simulink model "Q5_RMS"  (R2017b)
settings: Solver=VariableStepAuto  StartTime=0.0  StopTime=1000  RelTol=1e-3
libraries: dspstat3 x3
settings Model: Creator=YSNsec  LastModifiedBy=YSNsec
settings DataIOCC: ReturnWorkspaceOutputs=on
settings DebuggingCC: SFMachineParentedDataDiag=error
settings SFSimCC: SimUseLocalCustomCode=on
settings RTWCC: RTWUseLocalCustomCode=on

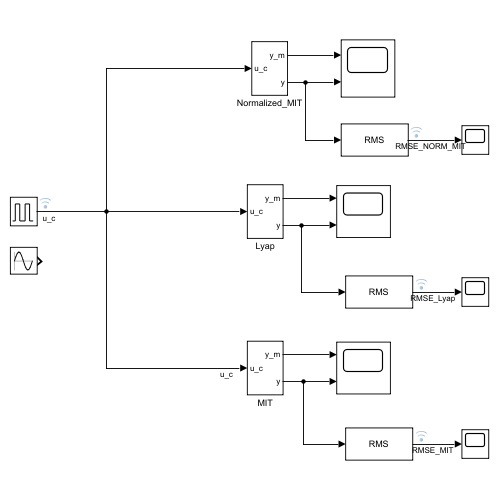
[thumbnail: Simulink's stored preview of the top-level diagram]
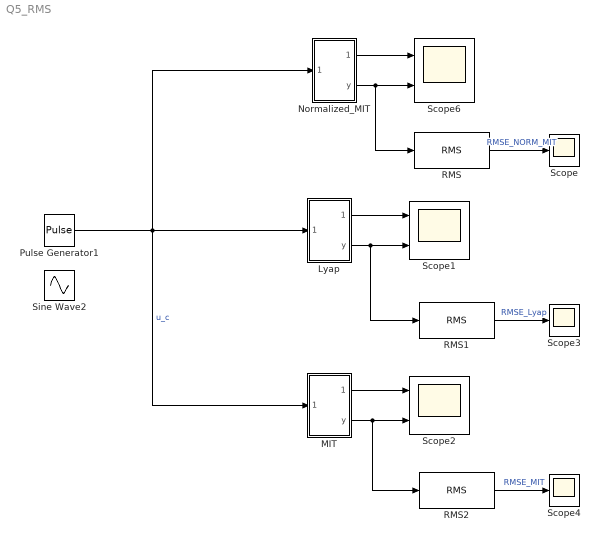
== system Q5_RMS ==
  Lyap : Subsystem
  MIT : Subsystem
  Normalized_MIT : Subsystem
  Pulse Generator1 : DiscretePulseGenerator  PulseType=Time based  Amplitude=10  Period=200  PulseWidth=50
  RMS : dspstat3/RMS  run=off  directionMode=Entire input  dimension=1  InputProcessing=Columns as channels (frame based)  reset_popup=None
  RMS1 : dspstat3/RMS  run=off  directionMode=Entire input  dimension=1  InputProcessing=Columns as channels (frame based)  reset_popup=None
  RMS2 : dspstat3/RMS  run=off  directionMode=Entire input  dimension=1  InputProcessing=Columns as channels (frame based)  reset_popup=None
  Scope : Scope
  Scope1 : Scope  NumInputPorts=2
  Scope2 : Scope  NumInputPorts=2
  Scope3 : Scope
  Scope4 : Scope
  Scope6 : Scope  NumInputPorts=2
  Sine Wave2 : Sin  Amplitude=10  Frequency=0.01  SampleTime=0
  wires:
  Normalized_MIT/1(y_m) -> Scope6/1
  Normalized_MIT/2(y) -> RMS/1, Scope6/2
  Lyap/1(y_m) -> Scope1/1
  Pulse Generator1/1 -> MIT/1(u_c), Lyap/1(u_c), Normalized_MIT/1(u_c)  "u_c"
  MIT/1(y_m) -> Scope2/1
  RMS/1 -> Scope/1  "RMSE_NORM_MIT"
  RMS1/1 -> Scope3/1  "RMSE_Lyap"
  Lyap/2(y) -> RMS1/1, Scope1/2
  RMS2/1 -> Scope4/1  "RMSE_MIT"
  MIT/2(y) -> RMS2/1, Scope2/2

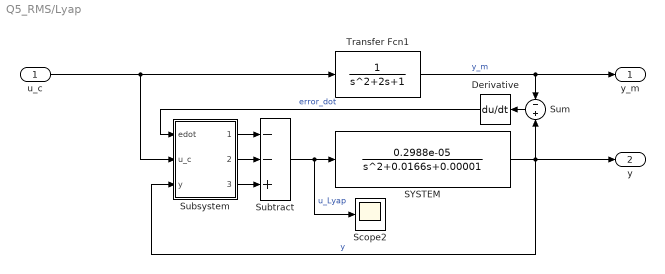
== system Q5_RMS/Lyap ==
  u_c : Inport
  Derivative : Derivative
  SYSTEM : TransferFcn  Numerator=0.2988e-05  Denominator=[1 0.0166 0.00001]
  Scope2 : Scope
  Subsystem : Subsystem
  Subtract : Sum  Inputs=--+
  Sum : Sum  Inputs=-|+
  Transfer Fcn1 : TransferFcn
  y_m : Outport
  y : Outport  Port=2
  wires:
  Subsystem/3(Theta1) -> Subtract/3
  SYSTEM/1 -> y/1, Subsystem/3(y), Sum/2  "y"
  Derivative/1 -> Subsystem/1(edot)  "error_dot"
  u_c/1 -> Subsystem/2(u_c), Transfer Fcn1/1
  Transfer Fcn1/1 -> y_m/1, Sum/1  "y_m"
  Subsystem/1(Theta3) -> Subtract/1
  Subsystem/2(Theta2) -> Subtract/2
  Subtract/1 -> SYSTEM/1, Scope2/1  "u_Lyap"
  Sum/1 -> Derivative/1

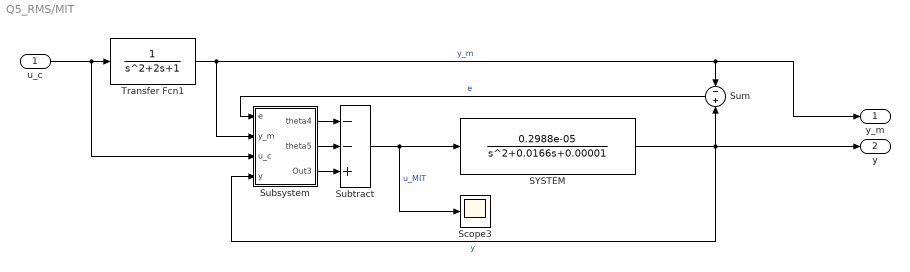
== system Q5_RMS/MIT ==
  u_c : Inport
  SYSTEM : TransferFcn  Numerator=0.2988e-05  Denominator=[1 0.0166 0.00001]
  Scope3 : Scope
  Subsystem : Subsystem
  Subtract : Sum  Inputs=--+
  Sum : Sum  Inputs=-|+
  Transfer Fcn1 : TransferFcn
  y_m : Outport
  y : Outport  Port=2
  wires:
  Subsystem/1(theta4) -> Subtract/1
  Sum/1 -> Subsystem/1(e)  "e"
  SYSTEM/1 -> y/1, Subsystem/4(y), Sum/2  "y"
  Subsystem/2(theta5) -> Subtract/2
  Transfer Fcn1/1 -> Subsystem/2(y_m), y_m/1, Sum/1  "y_m"
  u_c/1 -> Subsystem/3(u_c), Transfer Fcn1/1
  Subsystem/3(Out3) -> Subtract/3
  Subtract/1 -> SYSTEM/1, Scope3/1  "u_MIT"

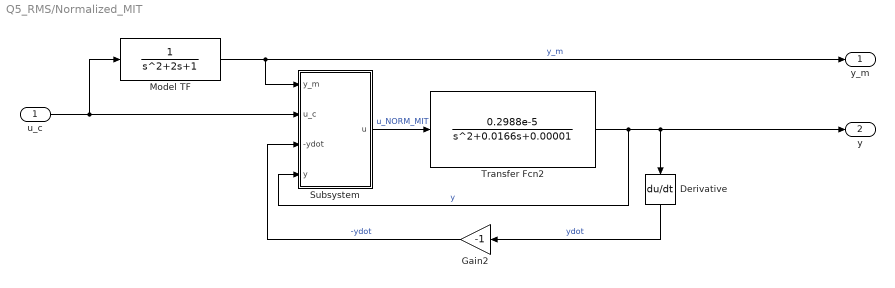
== system Q5_RMS/Normalized_MIT ==
  u_c : Inport
  Derivative : Derivative
  Gain2 : Gain  Gain=-1
  Model TF : TransferFcn  Numerator=1
  Subsystem : Subsystem
  Transfer Fcn2 : TransferFcn  Numerator=0.2988e-5  Denominator=[1 0.0166 0.00001]
  y_m : Outport
  y : Outport  Port=2
  wires:
  u_c/1 -> Model TF/1, Subsystem/2(u_c)
  Gain2/1 -> Subsystem/3(-ydot)  "-ydot"
  Model TF/1 -> y_m/1, Subsystem/1(y_m)  "y_m"
  Transfer Fcn2/1 -> y/1, Derivative/1, Subsystem/4(y)  "y"
  Derivative/1 -> Gain2/1  "ydot"
  Subsystem/1(u) -> Transfer Fcn2/1  "u_NORM_MIT"

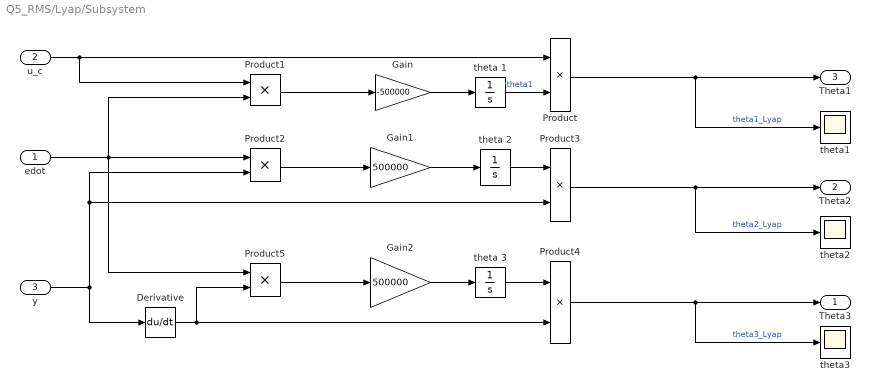
== system Q5_RMS/Lyap/Subsystem ==
  edot : Inport
  u_c : Inport  Port=2
  y : Inport  Port=3
  Derivative : Derivative
  Gain : Gain  Gain=-500000
  Gain1 : Gain  Gain=500000
  Gain2 : Gain  Gain=500000
  Product{,1..5} (6 alike) : Product
  theta 1 : Integrator
  theta 2 : Integrator
  theta 3 : Integrator
  theta1 : Scope
  theta2 : Scope
  theta3 : Scope
  Theta3 : Outport
  Theta2 : Outport  Port=2
  Theta1 : Outport  Port=3
  wires:
  Product3/1 -> theta2/1, Theta2/1  "theta2_Lyap"
  y/1 -> Product2/2, Product3/2, Derivative/1
  Derivative/1 -> Product5/2, Product4/2
  Product5/1 -> Gain2/1
  theta 1/1 -> Product/2  "theta1"
  Gain2/1 -> theta 3/1
  edot/1 -> Product1/2, Product5/1, Product2/1
  Gain1/1 -> theta 2/1
  Product1/1 -> Gain/1
  Product/1 -> Theta1/1, theta1/1  "theta1_Lyap"
  theta 3/1 -> Product4/1
  theta 2/1 -> Product3/1
  Product4/1 -> theta3/1, Theta3/1  "theta3_Lyap"
  Gain/1 -> theta 1/1
  Product2/1 -> Gain1/1
  u_c/1 -> Product1/1, Product/1

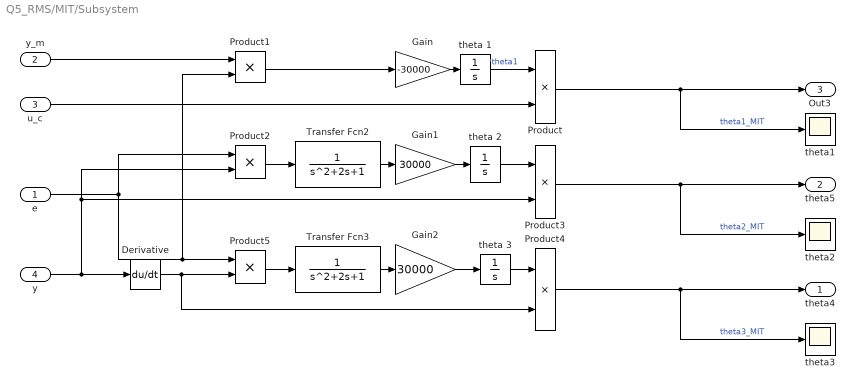
== system Q5_RMS/MIT/Subsystem ==
  e : Inport
  y_m : Inport  Port=2
  u_c : Inport  Port=3
  y : Inport  Port=4
  Derivative : Derivative
  Gain : Gain  Gain=-30000
  Gain1 : Gain  Gain=30000
  Gain2 : Gain  Gain=30000
  Product{,1..5} (6 alike) : Product
  Transfer Fcn2 : TransferFcn
  Transfer Fcn3 : TransferFcn
  theta 1 : Integrator
  theta 2 : Integrator
  theta 3 : Integrator
  theta1 : Scope
  theta2 : Scope
  theta3 : Scope
  theta4 : Outport
  theta5 : Outport  Port=2
  Out3 : Outport  Port=3
  wires:
  Product3/1 -> theta2/1, theta5/1  "theta2_MIT"
  y/1 -> Derivative/1, Product2/2, Product3/2
  Derivative/1 -> Product4/2, Product5/2
  Transfer Fcn3/1 -> Gain2/1
  theta 1/1 -> Product/1  "theta1"
  Gain2/1 -> theta 3/1
  e/1 -> Product1/2, Product5/1, Product2/1
  Gain1/1 -> theta 2/1
  Product1/1 -> Gain/1
  Product/1 -> theta1/1, Out3/1  "theta1_MIT"
  Product5/1 -> Transfer Fcn3/1
  theta 3/1 -> Product4/1
  theta 2/1 -> Product3/1
  Product4/1 -> theta3/1, theta4/1  "theta3_MIT"
  Product2/1 -> Transfer Fcn2/1
  Gain/1 -> theta 1/1
  Transfer Fcn2/1 -> Gain1/1
  y_m/1 -> Product1/1
  u_c/1 -> Product/2

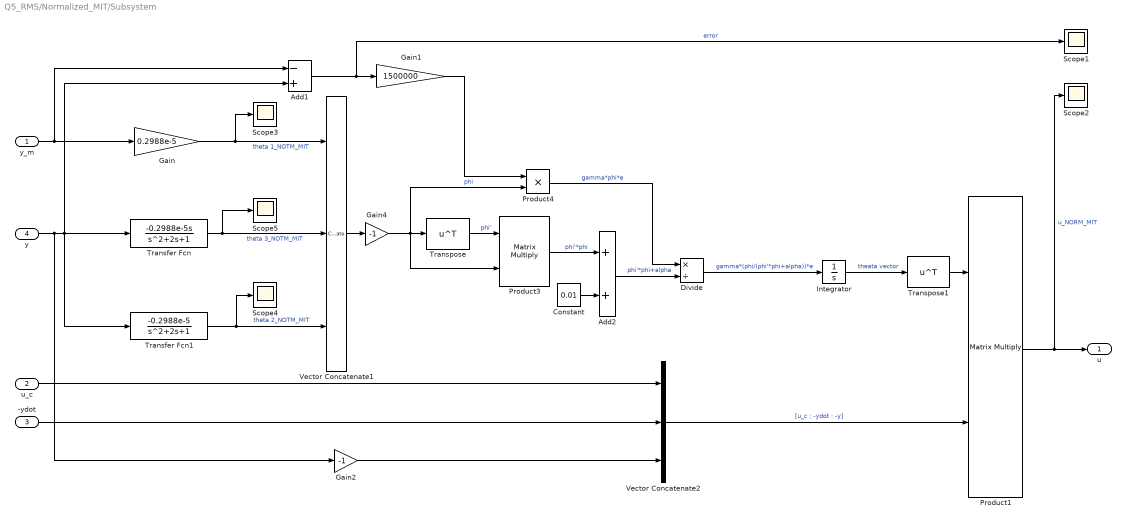
== system Q5_RMS/Normalized_MIT/Subsystem ==
  y_m : Inport
  u_c : Inport  Port=2
  -ydot : Inport  Port=3
  y : Inport  Port=4
  Add1 : Sum  Inputs=-+
  Add2 : Sum
  Constant : Constant  Value=0.01
  Divide : Product  Inputs=*/
  Gain : Gain  Gain=0.2988e-5
  Gain1 : Gain  Gain=1500000
  Gain2 : Gain  Gain=-1
  Gain4 : Gain  Gain=-1
  Integrator : Integrator
  Product1 : Product  Multiplication=Matrix(*)
  Product3 : Product  Multiplication=Matrix(*)
  Product4 : Product
  Scope{1..5} (5 alike) : Scope
  Transfer Fcn : TransferFcn  Numerator=[-0.2988e-5 0]
  Transfer Fcn1 : TransferFcn  Numerator=[-0.2988e-5]
  Transpose : Math  Operator=transpose  SaturateOnIntegerOverflow=on
  Transpose1 : Math  Operator=transpose  SaturateOnIntegerOverflow=on
  Vector Concatenate1 : Concatenate  NumInputs=3
  Vector Concatenate2 : Concatenate  NumInputs=3
  u : Outport
  wires:
  Gain/1 -> Scope3/1, Vector Concatenate1/1  "theta 1_NOTM_MIT"
  y/1 -> Transfer Fcn1/1, Transfer Fcn/1, Add1/2, Gain2/1
  Add1/1 -> Scope1/1, Gain1/1  "error"
  Product3/1 -> Add2/1  "phi'*phi"
  Constant/1 -> Add2/2
  Gain1/1 -> Product4/1
  Gain4/1 -> Product4/2, Product3/2, Transpose/1  "phi"
  Vector Concatenate1/1 -> Gain4/1
  Divide/1 -> Integrator/1  "gamma*(phi/(phi'*phi+alpha))*e"
  Transpose/1 -> Product3/1  "phi'"
  Add2/1 -> Divide/2  "phi'*phi+alpha"
  Transpose1/1 -> Product1/1
  Product1/1 -> u/1, Scope2/1  "u_NORM_MIT"
  Transfer Fcn/1 -> Scope5/1, Vector Concatenate1/2  "theta 3_NOTM_MIT"
  Integrator/1 -> Transpose1/1  "theata vector"
  Product4/1 -> Divide/1  "gamma*phi*e"
  Transfer Fcn1/1 -> Scope4/1, Vector Concatenate1/3  "theta 2_NOTM_MIT"
  y_m/1 -> Add1/1, Gain/1
  -ydot/1 -> Vector Concatenate2/2
  Vector Concatenate2/1 -> Product1/2  "[u_c ; -ydot : -y]"
  Gain2/1 -> Vector Concatenate2/3
  u_c/1 -> Vector Concatenate2/1
